simulink model "control_ms"  (Simulink 8.4)
settings: Solver=ode45  StartTime=0.0  StopTime=30  MaxStep=0.01  RelTol=1e-3
values from neighbouring files (symbols this model uses):
  A = XX    [codigo_Prac5.m]
  alpha = XX    [codigo_Prac5.m]
  beta_ctrl = XX    [codigo_Prac5.m]
  IncH2 = XX    [codigo_Prac5.m]
  IncQ = XX    [codigo_Prac5.m]
  k = As*sqrt(2*g)    [codigo_Prac5.m]
  K = XX    [codigo_Prac5.m]
  Kp_filter = XX    [codigo_Prac5.m]
  L = XX    [codigo_Prac5.m]
  Q = 2    [codigo_Prac5.m]
  T = tau    [codigo_Prac5.m]
  Td_filter = XX    [codigo_Prac5.m]
  Ti_filter = XX    [codigo_Prac5.m]
  x0_ini = [2*XX  XX]    [codigo_Prac5.m]
undefined symbols (not defined in the file or in its folder): Kc_filter
settings Model: Creator=carles  LastModifiedBy=win04  CovHtmlReporting=off
settings DebuggingCC: MaxConsecutiveZCsMsg=none  FcnCallInpInsideContextMsg=EnableAllAsWarning  FrameProcessingCompatibilityMsg=error

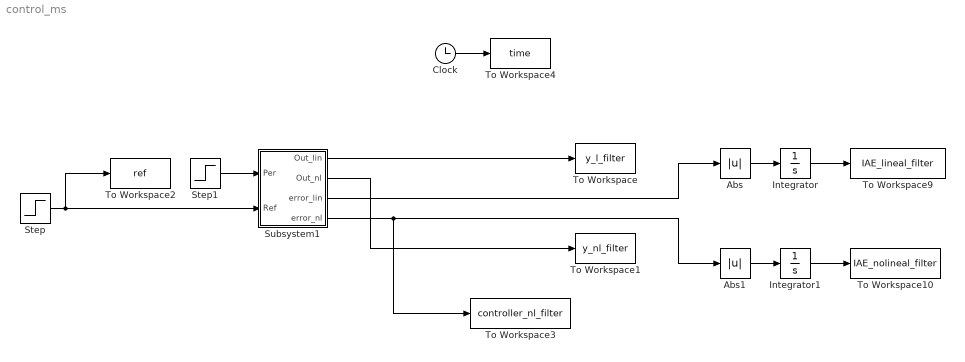
== system control_ms ==
  Abs : Abs
  Abs1 : Abs
  Clock : Clock
  Integrator : Integrator
  Integrator1 : Integrator
  Step : Step  Time=5  After=IncH2  SampleTime=0
  Step1 : Step  Time=20  After=IncQ  SampleTime=0
  Subsystem1 : Subsystem
  To Workspace : ToWorkspace  VariableName=y_l_filter  SampleTime=-1
  To Workspace1 : ToWorkspace  VariableName=y_nl_filter  SampleTime=-1
  To Workspace10 : ToWorkspace  VariableName=IAE_nolineal_filter  SampleTime=-1
  To Workspace2 : ToWorkspace  VariableName=ref  SampleTime=-1
  To Workspace3 : ToWorkspace  VariableName=controller_nl_filter  SampleTime=-1
  To Workspace4 : ToWorkspace  VariableName=time  SampleTime=-1
  To Workspace9 : ToWorkspace  VariableName=IAE_lineal_filter  SampleTime=-1
  wires:
  Step/1 -> To Workspace2/1, Subsystem1/2(Ref)
  Subsystem1/1(Out_lin) -> To Workspace/1
  Subsystem1/2(Out_nl) -> To Workspace1/1
  Step1/1 -> Subsystem1/1(Per)
  Abs/1 -> Integrator/1
  Integrator/1 -> To Workspace9/1
  Abs1/1 -> Integrator1/1
  Integrator1/1 -> To Workspace10/1
  Subsystem1/3(error_lin) -> Abs/1
  Subsystem1/4(error_nl) -> To Workspace3/1, Abs1/1
  Clock/1 -> To Workspace4/1

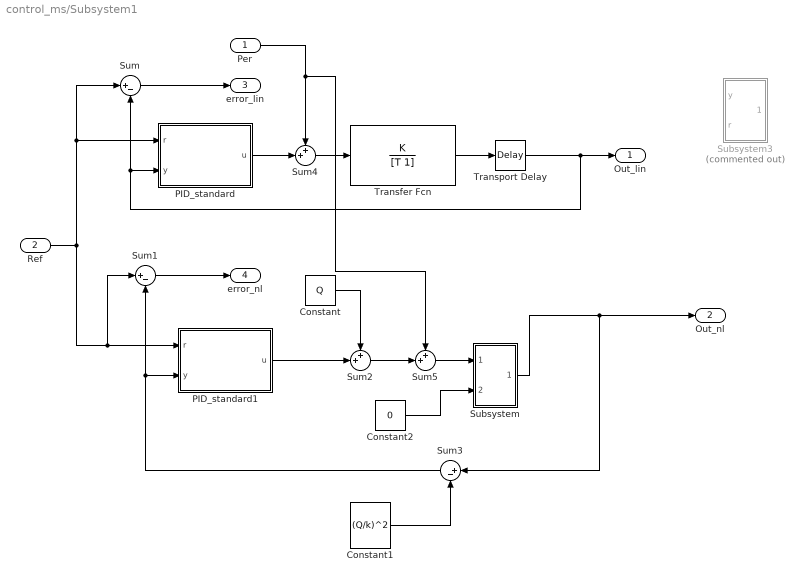
== system control_ms/Subsystem1 ==
  Per : Inport
  Ref : Inport  Port=2
  Constant : Constant  Value=Q
  Constant1 : Constant  Value=(Q/k)^2
  Constant2 : Constant  Value=0
  PID_standard : Subsystem
  PID_standard1 : Subsystem
  Subsystem : Subsystem
  Subsystem3 : Subsystem  Commented=on
  Sum : Sum  Inputs=|+-
  Sum1 : Sum  Inputs=|+-
  Sum2 : Sum  Inputs=++|
  Sum3 : Sum  Inputs=|+-
  Sum4 : Sum  Inputs=++|
  Sum5 : Sum  Inputs=++|
  Transfer Fcn : TransferFcn  Numerator=K  Denominator=[T 1]
  Transport Delay : TransportDelay  DelayTime=L
  Out_lin : Outport
  Out_nl : Outport  Port=2
  error_lin : Outport  Port=3
  error_nl : Outport  Port=4
  wires:
  Transport Delay/1 -> Sum/2, PID_standard/2(y), Out_lin/1
  Sum4/1 -> Transfer Fcn/1
  PID_standard1/1(u) -> Sum2/2
  Subsystem/1(Out2) -> Sum3/1, Out_nl/1
  Constant2/1 -> Subsystem/2(In2)
  Per/1 -> Sum5/1, Sum4/1
  Sum2/1 -> Sum5/2
  Constant/1 -> Sum2/1
  Constant1/1 -> Sum3/2
  Transfer Fcn/1 -> Transport Delay/1
  Sum3/1 -> PID_standard1/2(y), Sum1/2
  Sum5/1 -> Subsystem/1(In1)
  Ref/1 -> PID_standard1/1(r), Sum1/1, PID_standard/1(r), Sum/1
  Sum/1 -> error_lin/1
  PID_standard/1(u) -> Sum4/2
  Sum1/1 -> error_nl/1

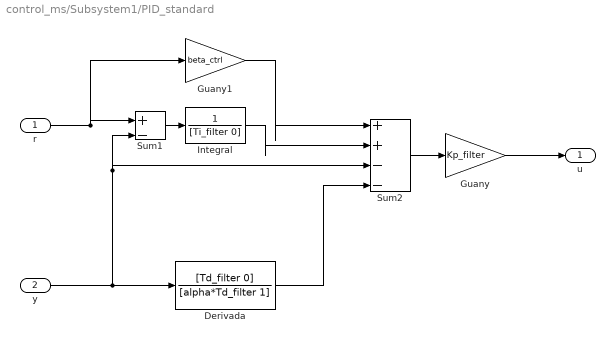
== system control_ms/Subsystem1/PID_standard ==
  r : Inport
  y : Inport  Port=2
  Derivada : TransferFcn  Numerator=[Td_filter 0]  Denominator=[alpha*Td_filter 1]
  Guany : Gain  Gain=Kp_filter
  Guany1 : Gain  Gain=beta_ctrl
  Integral : TransferFcn  Denominator=[Ti_filter 0]
  Sum1 : Sum  Inputs=|+-
  Sum2 : Sum  Inputs=|++--
  u : Outport
  wires:
  Guany/1 -> u/1
  Sum2/1 -> Guany/1
  r/1 -> Sum1/1, Guany1/1
  Guany1/1 -> Sum2/1
  Integral/1 -> Sum2/2
  y/1 -> Derivada/1, Sum2/3, Sum1/2
  Derivada/1 -> Sum2/4
  Sum1/1 -> Integral/1

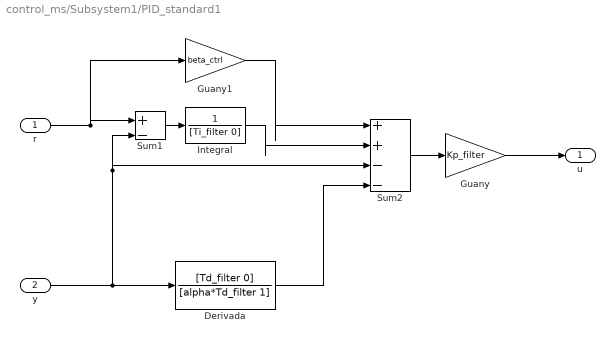
== system control_ms/Subsystem1/PID_standard1 ==
  r : Inport
  y : Inport  Port=2
  Derivada : TransferFcn  Numerator=[Td_filter 0]  Denominator=[alpha*Td_filter 1]
  Guany : Gain  Gain=Kp_filter
  Guany1 : Gain  Gain=beta_ctrl
  Integral : TransferFcn  Denominator=[Ti_filter 0]
  Sum1 : Sum  Inputs=|+-
  Sum2 : Sum  Inputs=|++--
  u : Outport
  wires:
  Guany/1 -> u/1
  Sum2/1 -> Guany/1
  r/1 -> Sum1/1, Guany1/1
  Guany1/1 -> Sum2/1
  Integral/1 -> Sum2/2
  y/1 -> Derivada/1, Sum2/3, Sum1/2
  Derivada/1 -> Sum2/4
  Sum1/1 -> Integral/1

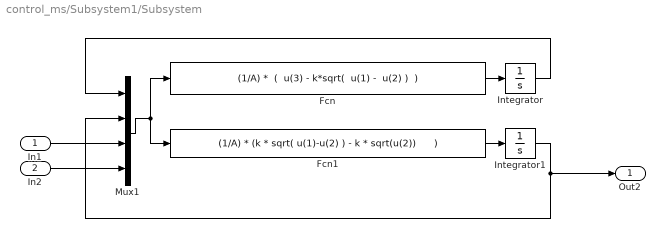
== system control_ms/Subsystem1/Subsystem ==
  In1 : Inport
  In2 : Inport  Port=2
  Fcn : Fcn  Expr="(1/A) *  (  u(3) - k*sqrt(  u(1) -  u(2) )  )"
  Fcn1 : Fcn  Expr="(1/A) * (k * sqrt( u(1)-u(2) ) - k * sqrt(u(2))      )"
  Integrator : Integrator  InitialCondition=x0_ini(1)
  Integrator1 : Integrator  InitialCondition=x0_ini(2)
  Mux1 : Mux
  Out2 : Outport
  wires:
  In1/1 -> Mux1/3
  In2/1 -> Mux1/4
  Integrator1/1 -> Out2/1, Mux1/2
  Integrator/1 -> Mux1/1
  Mux1/1 -> Fcn/1, Fcn1/1
  Fcn1/1 -> Integrator1/1
  Fcn/1 -> Integrator/1

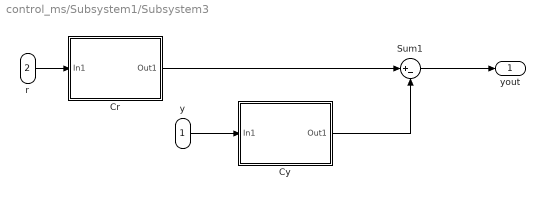
== system control_ms/Subsystem1/Subsystem3 ==
  y : Inport
  r : Inport  Port=2
  Cr : Subsystem
  Cy : Subsystem
  Sum1 : Sum  Inputs=|+-
  yout : Outport
  wires:
  y/1 -> Cy/1(In1)
  Sum1/1 -> yout/1
  Cy/1(Out1) -> Sum1/2
  Cr/1(Out1) -> Sum1/1
  r/1 -> Cr/1(In1)

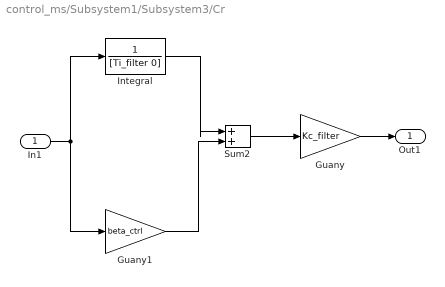
== system control_ms/Subsystem1/Subsystem3/Cr ==
  In1 : Inport
  Guany : Gain  Gain=Kc_filter
  Guany1 : Gain  Gain=beta_ctrl
  Integral : TransferFcn  Denominator=[Ti_filter 0]
  Sum2 : Sum  Inputs=|++
  Out1 : Outport
  wires:
  Guany/1 -> Out1/1
  Sum2/1 -> Guany/1
  Integral/1 -> Sum2/1
  In1/1 -> Guany1/1, Integral/1
  Guany1/1 -> Sum2/2

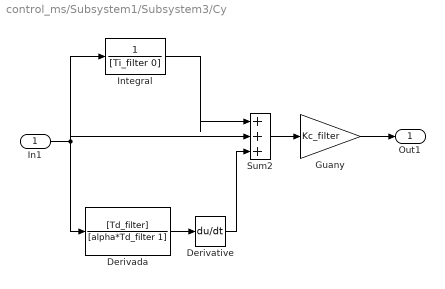
== system control_ms/Subsystem1/Subsystem3/Cy ==
  In1 : Inport
  Derivada : TransferFcn  Numerator=[Td_filter]  Denominator=[alpha*Td_filter 1]
  Derivative : Derivative
  Guany : Gain  Gain=Kc_filter
  Integral : TransferFcn  Denominator=[Ti_filter 0]
  Sum2 : Sum  Inputs=|+++
  Out1 : Outport
  wires:
  Guany/1 -> Out1/1
  Sum2/1 -> Guany/1
  Integral/1 -> Sum2/1
  In1/1 -> Sum2/2, Derivada/1, Integral/1
  Derivada/1 -> Derivative/1
  Derivative/1 -> Sum2/3
